simulink model "PID"  (R2014a)
settings: Solver=ode45  StartTime=0.0  StopTime=10.0  RelTol=1e-3
settings Model: Creator=pengpeng  LastModifiedBy=pengpeng

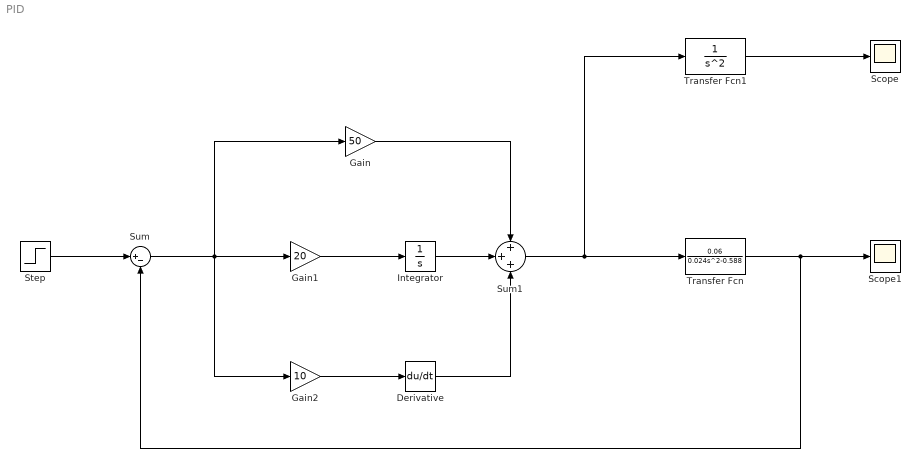
== system PID ==
  Derivative : Derivative
  Gain : Gain  Gain=50
  Gain1 : Gain  Gain=20
  Gain2 : Gain  Gain=10
  Integrator : Integrator
  Scope : Scope
  Scope1 : Scope
  Step : Step  Time=0  SampleTime=0
  Sum : Sum  Inputs=|+-
  Sum1 : Sum  Inputs=+++
  Transfer Fcn : TransferFcn  Numerator=[0.06]  Denominator=[0.024 0 -0.588]
  Transfer Fcn1 : TransferFcn  Denominator=[1 0 0]
  wires:
  Step/1 -> Sum/1
  Sum/1 -> Gain2/1, Gain/1, Gain1/1
  Gain1/1 -> Integrator/1
  Integrator/1 -> Sum1/2
  Gain/1 -> Sum1/1
  Gain2/1 -> Derivative/1
  Derivative/1 -> Sum1/3
  Sum1/1 -> Transfer Fcn1/1, Transfer Fcn/1
  Transfer Fcn/1 -> Sum/2, Scope1/1
  Transfer Fcn1/1 -> Scope/1
